simulink model "testTemp"  (R2013a)
settings: Solver=ode4  StartTime=0.0  StopTime=100  FixedStep=1e-3  RelTol=1e-5
values from neighbouring files (symbols this model uses):
  F0_ER = F_initial    [initHybrid.m]    (also in initMV.m; init_MVM.m)
  nStroke = 2    [Init8RTFLEX68D.m]
  p0_AR = p_acool    [initHybrid.m]    (also in initMV.m; init_MVM.m)
  p0_ER = p_exh_init    [initHybrid.m]    (also in initMV.m; init_MVM.m)
  T0_AR = T_acool    [initHybrid.m]    (also in initMV.m; init_MVM.m)
  T0_ER = 800    [initHybrid.m]    (also in initMV.m; init_MVM.m)
undefined symbols (not defined in the file): generators
libraries: simulink x1, EngineSystemSubmodelVer1_0 x1
settings Model: Creator=yum  LastModifiedBy=yum
settings DataIOCC: InspectSignalLogs=on

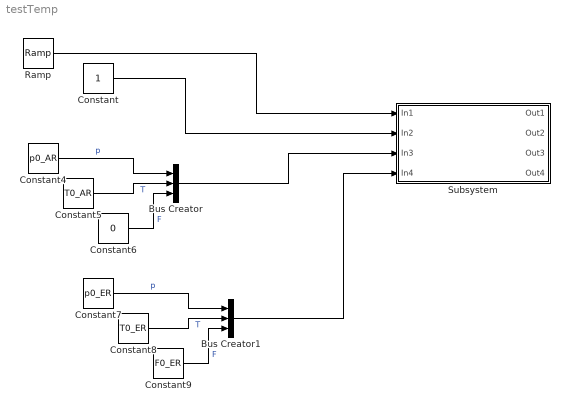
== system testTemp ==
  Bus Creator : BusCreator  Inputs=3
  Bus Creator1 : BusCreator  Inputs=3
  Constant : Constant
  Constant4 : Constant  Value=p0_AR
  Constant5 : Constant  Value=T0_AR
  Constant6 : Constant  Value=0
  Constant7 : Constant  Value=p0_ER
  Constant8 : Constant  Value=T0_ER
  Constant9 : Constant  Value=F0_ER
  Ramp : simulink/Sources/Ramp  slope=1  start=0  X0=0
  Subsystem : Subsystem  mask{genset=generators(1)}
      mask prompts: genset "Param"
  wires:
  Constant4/1 -> Bus Creator/1  "p"
  Constant5/1 -> Bus Creator/2  "T"
  Constant6/1 -> Bus Creator/3  "F"
  Constant7/1 -> Bus Creator1/1  "p"
  Constant8/1 -> Bus Creator1/2  "T"
  Constant9/1 -> Bus Creator1/3  "F"
  Ramp/1 -> Subsystem/1(In1)
  Constant/1 -> Subsystem/2(In2)
  Bus Creator/1 -> Subsystem/3(In3)
  Bus Creator1/1 -> Subsystem/4(In4)

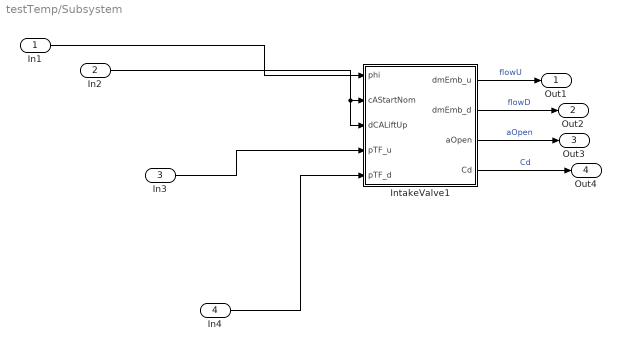
== system testTemp/Subsystem ==
  In1 : Inport
  In2 : Inport  Port=2
  In3 : Inport  Port=3
  In4 : Inport  Port=4
  IntakeValve1 : Subsystem  mask{fs=genset.eng.fs, nStroke=int8(nStroke), cAVVUpRef=genset.eng.cAVVUpRef, cAVVDownRef=genset.eng.cAVVDownRef, liftUpRef=genset.eng.liftUpRef, liftDownRef=genset.eng.liftDownRef, cAStartRef=genset.eng.intakeStartCARef, dCALiftUp=genset.eng.dCAIntakeLiftUpRef, dCALiftDown=genset.eng.dCAIntakeLiftDown, dCALiftTopRef=genset.eng.dCAIntakeLiftTopRef, liftMax=genset.eng.intakeLiftMaxRef, Dv=genset.eng.intakeDV, beta=genset.eng.intakeBeta, w=genset.eng.intakeW, Dp=genset.eng.intakeDp, Ds=genset.eng.intakeDs}
      mask prompts: fs "Stoichiometric fuel-air equivalent ratio"; nStroke "Number of stroke"; cAVVUpRef "Crank angle array for opening [deg]"; cAVVDownRef "Crank angle array for closing [deg]"; liftUpRef "Normalized lift array for opening (0~1)"; liftDownRef "Normalized lift array for closing (0~1)"; cAStartRef "Nominal crank angle at start of valve lif [deg]"; dCALiftUp "Nominal duration of crank angle for valve opening [deg]"; dCALiftDown "Nominal duration of crank angle for valve closing [deg]"; dCALiftTopRef "Nominal duration of crank angle for valve open [deg]"; liftMax "Maximum valve lift [m]"; Dv "Valve head diameter [m]"; beta "Seat angle [rad]"; w "Valve seat width [m]"; Dp "Inner seat diameter [m]"; Ds "Stem diameter [m]"
      mask TypeOptions fs: IdealNozzle/fs
      mask TypeOptions nStroke: S-Function/nStroke
      mask TypeOptions cAVVUpRef: S-Function/cAVVUpRef
      mask TypeOptions cAVVDownRef: S-Function/cAVVDownRef
      mask TypeOptions liftUpRef: S-Function/liftUpRef
      mask TypeOptions liftDownRef: S-Function/liftDownRef
      mask TypeOptions cAStartRef: S-Function/cAStartRef
      mask TypeOptions dCALiftUp: S-Function/dCALiftUp
      mask TypeOptions dCALiftDown: S-Function/dCALiftDown
      mask TypeOptions dCALiftTopRef: S-Function/dCALiftTopRef
      mask TypeOptions liftMax: S-Function/liftMax
      mask TypeOptions Dv: S-Function1/Dv
      mask TypeOptions beta: S-Function1/beta
      mask TypeOptions w: S-Function1/w
      mask TypeOptions Dp: S-Function1/Dp
      mask TypeOptions Ds: S-Function1/Ds
  Out1 : Outport
  Out2 : Outport  Port=2
  Out3 : Outport  Port=3
  Out4 : Outport  Port=4
  wires:
  In4/1 -> IntakeValve1/5(pTF_d)
  In3/1 -> IntakeValve1/4(pTF_u)
  IntakeValve1/4(Cd) -> Out4/1  "Cd"
  In1/1 -> IntakeValve1/1(phi)
  IntakeValve1/3(aOpen) -> Out3/1  "aOpen"
  IntakeValve1/1(dmEmb_u) -> Out1/1  "flowU"
  IntakeValve1/2(dmEmb_d) -> Out2/1  "flowD"
  In2/1 -> IntakeValve1/3(dCALiftUp), IntakeValve1/2(cAStartNom)

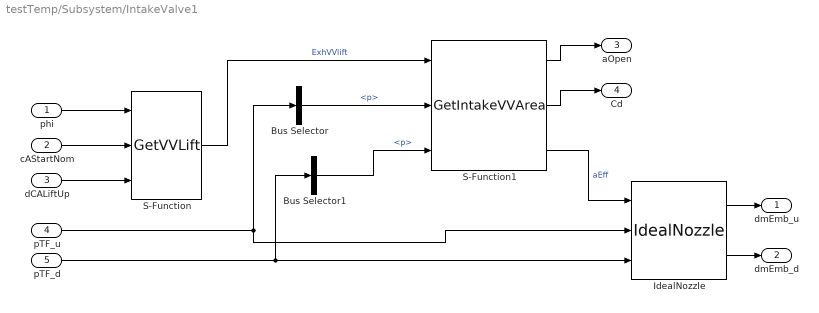
== system testTemp/Subsystem/IntakeValve1 ==
  phi : Inport
  cAStartNom : Inport  Port=2
  dCALiftUp : Inport  Port=3
  pTF_u : Inport  Port=4
  pTF_d : Inport  Port=5
  Bus Selector : BusSelector  OutputSignals=p
  Bus Selector1 : BusSelector  OutputSignals=p
  IdealNozzle : EngineSystemSubmodelVer1_0/IdealNozzle  fs=fs
  S-Function : S-Function  FunctionName=GetVVLift  Parameters=nStroke,liftMax,cAStartRef,dCALiftUp,dCALiftDown,dCALiftTopRef,cAVVUpRef,cAVVDownRef,liftUpRef,liftDownRef  EnableBusSupport=off  mask{nStroke=nStroke, liftMax=liftMax, cAStartRef=cAStartRef, dCALiftUp=dCALiftUp, dCALiftDown=dCALiftDown, dCALiftTopRef=dCALiftTopRef, cAVVUpRef=cAVVUpRef, cAVVDownRef=cAVVDownRef, liftUpRef=liftUpRef, liftDownRef=liftDownRef}
      mask prompts: nStroke "Number of stroke"; liftMax "Maximum valve lift [m]"; cAStartRef "Crank angle at the beginning of valve lift [deg]"; dCALiftUp "Duration for valve lifting [deg]"; dCALiftDown "Duration for valve closing [deg]"; dCALiftTopRef "Duration for valve fully opened [deg]"; cAVVUpRef "Crank angle array reference for valve opening [deg]"; cAVVDownRef "Crank angle array reference for valve closing [deg]"; liftUpRef "Normalized lift reference for valve opening (0~1)"; liftDownRef "Normalized lift reference for valve closing (0~1)"
  S-Function1 : S-Function  FunctionName=GetIntakeVVArea  Parameters=Dv,beta,w,Dp,Ds  EnableBusSupport=off  mask{Dv=Dv, beta=beta, w=w, Dp=Dp, Ds=Ds}
      mask prompts: Dv "Valve head diameter"; beta "Seat angle"; w "Valve seat width"; Dp "Inner seat diameter"; Ds "Stem diameter"
  dmEmb_u : Outport
  dmEmb_d : Outport  Port=2
  aOpen : Outport  Port=3
  Cd : Outport  Port=4
  wires:
  S-Function1/2 -> Cd/1
  S-Function1/1 -> aOpen/1
  S-Function1/3 -> IdealNozzle/1  "aEff"
  dCALiftUp/1 -> S-Function/3
  cAStartNom/1 -> S-Function/2
  phi/1 -> S-Function/1
  IdealNozzle/1 -> dmEmb_u/1
  IdealNozzle/2 -> dmEmb_d/1
  pTF_u/1 -> IdealNozzle/2, Bus Selector/1
  pTF_d/1 -> Bus Selector1/1, IdealNozzle/3
  S-Function/1 -> S-Function1/1  "ExhVVlift"
  Bus Selector/1 -> S-Function1/2  "<p>"
  Bus Selector1/1 -> S-Function1/3  "<p>"
